simulink model "prob8"  (R2020b)
settings: Solver=VariableStepAuto  StartTime=0.0  StopTime=10.0  RelTol=1e-3
settings Model: Creator=Nitin  LastModifiedBy=Nitin

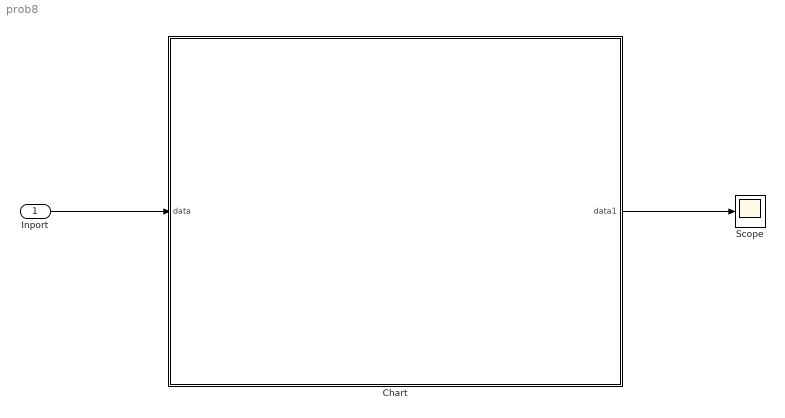
== system prob8 ==
  Inport : Inport
  Chart : Stateflow chart  TreatAsAtomicUnit=on
  Scope : Scope
  wires:
  Inport/1 -> Chart/1(data)
  Chart/1(data1) -> Scope/1

== stateflow chart prob8/Chart ==
  state On
    entry:
    power=1;
    state ground
      entry:
      floor=0;
    state first
      entry:
      floor=1;
    state second
      entry:
      floor=2;
    state third
      entry:
      floor=3;
    state fourth
      entry:
      floor=4;
    state fifth
      entry:
      floor=5;
    (default) -> ground
    second -> third [order 2] : [floor==3]
    ground -> first : [floor==1]
    third -> fourth [order 2] : [floor==4]
    fourth -> fifth [order 2] : [floor==5]
    first -> second [order 2] : [floor==2]
    third -> second [order 1] : [floor==2]
    second -> first [order 1] : [floor==1]
    fifth -> fourth : [floor==4]
    fourth -> third [order 1] : [floor==3]
    first -> ground [order 1] : [floor==0]
  state Off
    entry:
    power=0;
  (default) -> On
  On -> Off : [power==0]
  Off -> On : [power==1]
  data: data input; data1 output; floor local; power local
